simulink model "SWC_HALOUT_type"  (R2021b)
settings: Solver=FixedStepDiscrete  StartTime=0.0  StopTime=10.0  FixedStep=0.005  RelTol=1e-3
values from neighbouring files (symbols this model uses):
  DTC_10020B = Simulink.Parameter    [DTC_Constant_Definition.m]
  DTC_10020C = Simulink.Parameter    [DTC_Constant_Definition.m]
  DTC_10020D = Simulink.Parameter    [DTC_Constant_Definition.m]
  DTC_10020E = Simulink.Parameter    [DTC_Constant_Definition.m]
  DTC_100210 = Simulink.Parameter    [DTC_Constant_Definition.m]
  DTC_100211 = Simulink.Parameter    [DTC_Constant_Definition.m]
  DTC_100212 = Simulink.Parameter    [DTC_Constant_Definition.m]
  DTC_100213 = Simulink.Parameter    [DTC_Constant_Definition.m]
  DTC_100214 = Simulink.Parameter    [DTC_Constant_Definition.m]
  DTC_100215 = Simulink.Parameter    [DTC_Constant_Definition.m]
  DTC_100216 = Simulink.Parameter    [DTC_Constant_Definition.m]
  DTC_100217 = Simulink.Parameter    [DTC_Constant_Definition.m]
  DTC_100218 = Simulink.Parameter    [DTC_Constant_Definition.m]
  DTC_100219 = Simulink.Parameter    [DTC_Constant_Definition.m]
  DTC_10021A = Simulink.Parameter    [DTC_Constant_Definition.m]
  DTC_10021B = Simulink.Parameter    [DTC_Constant_Definition.m]
  DTC_10021C = Simulink.Parameter    [DTC_Constant_Definition.m]
  DTC_10021D = Simulink.Parameter    [DTC_Constant_Definition.m]
  DTC_10021E = Simulink.Parameter    [DTC_Constant_Definition.m]
  DTC_100220 = Simulink.Parameter    [DTC_Constant_Definition.m]
  DTC_100221 = Simulink.Parameter    [DTC_Constant_Definition.m]
  DTC_100223 = Simulink.Parameter    [DTC_Constant_Definition.m]
  DTC_100224 = Simulink.Parameter    [DTC_Constant_Definition.m]
  DTC_100225 = Simulink.Parameter    [DTC_Constant_Definition.m]
  DTC_100226 = Simulink.Parameter    [DTC_Constant_Definition.m]
  DTC_100227 = Simulink.Parameter    [DTC_Constant_Definition.m]
  DTC_100242 = Simulink.Parameter    [DTC_Constant_Definition.m]
  DTC_100243 = Simulink.Parameter    [DTC_Constant_Definition.m]
  DTC_100244 = Simulink.Parameter    [DTC_Constant_Definition.m]
  DTC_100247 = Simulink.Parameter    [DTC_Constant_Definition.m]
  DTC_100248 = Simulink.Parameter    [DTC_Constant_Definition.m]
  DTC_100249 = Simulink.Parameter    [DTC_Constant_Definition.m]
  DTC_100250 = Simulink.Parameter    [DTC_Constant_Definition.m]
  DTC_100251 = Simulink.Parameter    [DTC_Constant_Definition.m]
  DTC_100252 = Simulink.Parameter    [DTC_Constant_Definition.m]
  DTC_100A10 = Simulink.Parameter    [DTC_Constant_Definition.m]
  DTC_100A12 = Simulink.Parameter    [DTC_Constant_Definition.m]
  DTC_100A16 = Simulink.Parameter    [DTC_Constant_Definition.m]
  DTC_100A17 = Simulink.Parameter    [DTC_Constant_Definition.m]
  DTC_100A18 = Simulink.Parameter    [DTC_Constant_Definition.m]
  DTC_100A19 = Simulink.Parameter    [DTC_Constant_Definition.m]
  DTC_500B01 = Simulink.Parameter    [DTC_Constant_Definition.m]
  DTC_500B02 = Simulink.Parameter    [DTC_Constant_Definition.m]
  DTC_500B03 = Simulink.Parameter    [DTC_Constant_Definition.m]
  DTC_500B04 = Simulink.Parameter    [DTC_Constant_Definition.m]
  DTC_500B05 = Simulink.Parameter    [DTC_Constant_Definition.m]
  DTC_500B06 = Simulink.Parameter    [DTC_Constant_Definition.m]
  DTC_500B07 = Simulink.Parameter    [DTC_Constant_Definition.m]
  DTC_500B08 = Simulink.Parameter    [DTC_Constant_Definition.m]
  DTC_500B09 = Simulink.Parameter    [DTC_Constant_Definition.m]
  DTC_500B0A = Simulink.Parameter    [DTC_Constant_Definition.m]
  DTC_500B0B = Simulink.Parameter    [DTC_Constant_Definition.m]
  DTC_500B0C = Simulink.Parameter    [DTC_Constant_Definition.m]
  DTC_500B0D = Simulink.Parameter    [DTC_Constant_Definition.m]
  DTC_500B0E = Simulink.Parameter    [DTC_Constant_Definition.m]
  DTC_500B0F = Simulink.Parameter    [DTC_Constant_Definition.m]
  DTC_500B10 = Simulink.Parameter    [DTC_Constant_Definition.m]
  DTC_90021F = Simulink.Parameter    [DTC_Constant_Definition.m]
  DTC_90022F = Simulink.Parameter    [DTC_Constant_Definition.m]
  DTC_900253 = Simulink.Parameter    [DTC_Constant_Definition.m]
  DTC_900254 = Simulink.Parameter    [DTC_Constant_Definition.m]
  DTC_900301 = Simulink.Parameter    [DTC_Constant_Definition.m]
  DTC_900302 = Simulink.Parameter    [DTC_Constant_Definition.m]
  DTC_900303 = Simulink.Parameter    [DTC_Constant_Definition.m]
  DTC_900304 = Simulink.Parameter    [DTC_Constant_Definition.m]
  DTC_900305 = Simulink.Parameter    [DTC_Constant_Definition.m]
  DTC_900909 = Simulink.Parameter    [DTC_Constant_Definition.m]
  DTC_90090A = Simulink.Parameter    [DTC_Constant_Definition.m]
  DTC_90090B = Simulink.Parameter    [DTC_Constant_Definition.m]
  DTC_90090C = Simulink.Parameter    [DTC_Constant_Definition.m]
  DTC_90090D = Simulink.Parameter    [DTC_Constant_Definition.m]
  DTC_90090E = Simulink.Parameter    [DTC_Constant_Definition.m]
  DTC_90090F = Simulink.Parameter    [DTC_Constant_Definition.m]
  DTC_900910 = Simulink.Parameter    [DTC_Constant_Definition.m]
  DTC_900911 = Simulink.Parameter    [DTC_Constant_Definition.m]
  DTC_900912 = Simulink.Parameter    [DTC_Constant_Definition.m]
  DTC_900913 = Simulink.Parameter    [DTC_Constant_Definition.m]
  DTC_900914 = Simulink.Parameter    [DTC_Constant_Definition.m]
  DTC_C0288F = Simulink.Parameter    [DTC_Constant_Definition.m]
  DTC_C0378F = Simulink.Parameter    [DTC_Constant_Definition.m]
  DTC_C0468F = Simulink.Parameter    [DTC_Constant_Definition.m]
  DTC_C0558F = Simulink.Parameter    [DTC_Constant_Definition.m]
  DTC_C0648F = Simulink.Parameter    [DTC_Constant_Definition.m]
  DTC_C0808F = Simulink.Parameter    [DTC_Constant_Definition.m]
  DTC_D00201 = Simulink.Parameter    [DTC_Constant_Definition.m]
  DTC_D00202 = Simulink.Parameter    [DTC_Constant_Definition.m]
  DTC_D00203 = Simulink.Parameter    [DTC_Constant_Definition.m]
  DTC_D00204 = Simulink.Parameter    [DTC_Constant_Definition.m]
  DTC_D00205 = Simulink.Parameter    [DTC_Constant_Definition.m]
  DTC_D00206 = Simulink.Parameter    [DTC_Constant_Definition.m]
  DTC_D00207 = Simulink.Parameter    [DTC_Constant_Definition.m]
  DTC_D00208 = Simulink.Parameter    [DTC_Constant_Definition.m]
  DTC_D00209 = Simulink.Parameter    [DTC_Constant_Definition.m]
  DTC_D0020A = Simulink.Parameter    [DTC_Constant_Definition.m]
  DTC_D00228 = Simulink.Parameter    [DTC_Constant_Definition.m]
  DTC_D00229 = Simulink.Parameter    [DTC_Constant_Definition.m]
  DTC_D0022A = Simulink.Parameter    [DTC_Constant_Definition.m]
  DTC_D0022B = Simulink.Parameter    [DTC_Constant_Definition.m]
  DTC_D0022C = Simulink.Parameter    [DTC_Constant_Definition.m]
  DTC_D0022D = Simulink.Parameter    [DTC_Constant_Definition.m]
  DTC_D00230 = Simulink.Parameter    [DTC_Constant_Definition.m]
  DTC_D00231 = Simulink.Parameter    [DTC_Constant_Definition.m]
  DTC_D00232 = Simulink.Parameter    [DTC_Constant_Definition.m]
  DTC_D00234 = Simulink.Parameter    [DTC_Constant_Definition.m]
  DTC_D00235 = Simulink.Parameter    [DTC_Constant_Definition.m]
  DTC_D00236 = Simulink.Parameter    [DTC_Constant_Definition.m]
  DTC_D00237 = Simulink.Parameter    [DTC_Constant_Definition.m]
  DTC_D00238 = Simulink.Parameter    [DTC_Constant_Definition.m]
  DTC_D0023A = Simulink.Parameter    [DTC_Constant_Definition.m]
  DTC_D0023B = Simulink.Parameter    [DTC_Constant_Definition.m]
  DTC_D0023C = Simulink.Parameter    [DTC_Constant_Definition.m]
  DTC_D0023D = Simulink.Parameter    [DTC_Constant_Definition.m]
  DTC_D0023E = Simulink.Parameter    [DTC_Constant_Definition.m]
  DTC_D00240 = Simulink.Parameter    [DTC_Constant_Definition.m]
  DTC_D00241 = Simulink.Parameter    [DTC_Constant_Definition.m]
undefined symbols (not defined in the file or in its folder): DIDLen_APPD, DIDLen_APPE, DIDLen_APPPedalZP, DIDLen_APSFunConfig, DIDLen_AutoLock, DIDLen_AutoWipHSpdEN, DIDLen_CALID, DIDLen_CDEODT, DIDLen_CLRDIST, DIDLen_DKCBLESta, DIDLen_DKCKey, DIDLen_DKCSta, DIDLen_DoorNFCAnchorSta, DIDLen_DRLDis, DIDLen_DynoMode, DIDLen_ECUNAME, DIDLen_FDDKCCoordXY, DIDLen_FMHTimer, DIDLen_LFLowPresThre, DIDLen_LFSensorID, DIDLen_LIDAAnchorSta, DIDLen_LRLowPresThre, DIDLen_LRSensorID, DIDLen_MILDIST, DIDLen_NUMPSATRIPSFLTMEMCLR, DIDLen_NVMPedalZP, DIDLen_OBDReq, DIDLen_ODOMETER, DIDLen_PKE, DIDLen_ProtocolId, DIDLen_PSA, DIDLen_QTYPSATRIPS, DIDLen_RFLowPresThre, DIDLen_RFSensorID, DIDLen_RRLowPresThre, DIDLen_RRSensorID, DIDLen_RUNTM, DIDLen_SensorMode, DIDLen_TestGroup, DIDLen_TireSize, DIDLen_TPMSLearnSta, DIDLen_UIDSta, DIDLen_USSConfig, DIDLen_UWBAnchorSta, DIDLen_VIN, DIDLen_VSS, DIDLen_WhlPres, DIDLen_WhlSensorBattSta, DIDLen_WhlTmp, DIDLen_WipRLSCmdCutFilter, DIDLen_WipRLSCmdHoldFilter, DIDLen_XWDMode, DIDNum_APPD, DIDNum_APPE, DIDNum_APPPedalZP, DIDNum_APSFunConfig, DIDNum_AutoLock, DIDNum_AutoWipHSpdEN, DIDNum_CALID, DIDNum_CDEODT ... (+281)
libraries: simulink x213, FVT_lib x160, hdlsllib x6, hcu_lib x5, halout x1
(part 9 of 9)

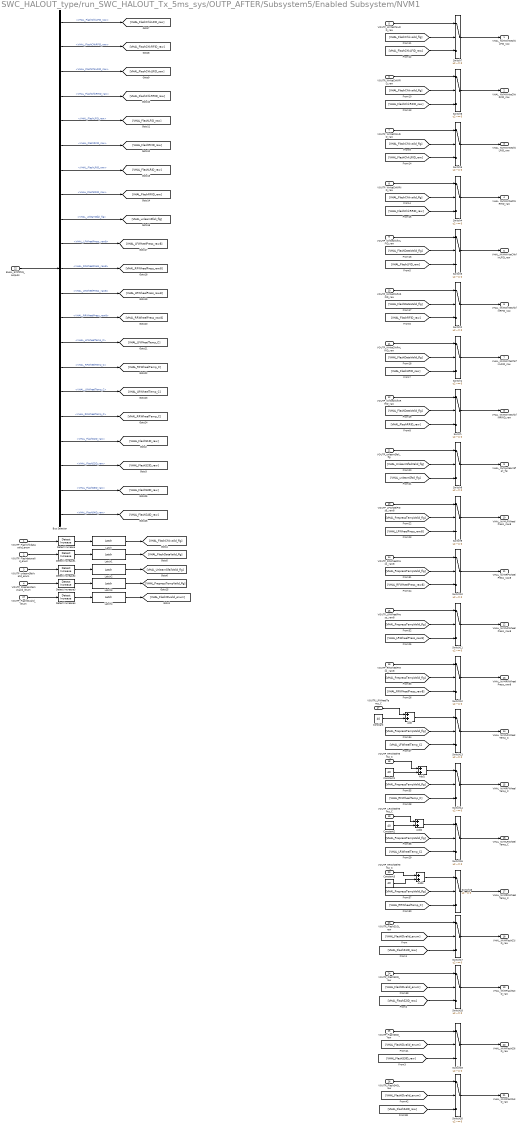
== system SWC_HALOUT_type/run_SWC_HALOUT_Tx_5ms_sys/OUTP_AFTER/Subsystem5/Enabled Subsystem/NVM1 ==
  VOUTP_Flashchkdatavalid_enum : Inport
  VOUTP_Flashdatavalid_enum : Inport  Port=2
  VOUTP_unlearnSfailvalid_enum : Inport  Port=3
  VOUTP_Prepresstempvalid_enum : Inport  Port=4
  VOUTP_WriteChkLFID_raw : Inport  Port=5
  VOUTP_WriteChkRFID_raw : Inport  Port=6
  VOUTP_WriteChkLRID_raw : Inport  Port=7
  VOUTP_WriteChkRRID_raw : Inport  Port=8
  VOUTP_WriteChkfinLFID_raw : Inport  Port=9
  VOUTP_WriteChkfinRFID_raw : Inport  Port=10
  VOUTP_WriteChkfinLRID_raw : Inport  Port=11
  VOUTP_WriteChkfinRRID_raw : Inport  Port=12
  VOUTP_LFWheelPress_raw8 : Inport  Port=13
  VOUTP_RFWheelPress_raw8 : Inport  Port=14
  VOUTP_LRWheelPress_raw8 : Inport  Port=15
  VOUTP_RRWheelPress_raw8 : Inport  Port=16
  VOUTP_LFWheelTemp_C : Inport  Port=17
  VOUTP_RFWheelTemp_C : Inport  Port=18
  VOUTP_LRWheelTemp_C : Inport  Port=19
  VOUTP_RRWheelTemp_C : Inport  Port=20
  VOUTP_unlearnSfali_flg : Inport  Port=21
  BHAL_SYSTPMS_outputs : Inport  Port=22
  VOUTP_FlashS1ID_raw : Inport  Port=23
  VOUTP_FlashS2ID_raw : Inport  Port=24
  VOUTP_FlashS3ID_raw : Inport  Port=25
  VOUTP_FlashS4ID_raw : Inport  Port=26
  VOUTP_FlashIDvalid_enum : Inport  Port=27
  Add{,1..3} (4 alike) : Sum
  Bus Selector : BusSelector  OutputSignals=VHAL_FlashChkLFID_raw,VHAL_FlashChkRFID_raw,VHAL_FlashChkLRID_raw,VHAL_FlashChkRRID_raw,VHAL_FlashLFID_raw,VHAL_FlashRFID_raw,VHAL_FlashLRID_raw,VHAL_FlashRRID_raw,VHAL_unlearnSfali_flg,VHAL_LFWheelPress_raw8,VHAL_RFWheelPress_raw8,VHAL_LRWheelPress_raw8,VHAL_RRWheelPress_raw8,VHAL_LFWheelTemp_C,VHAL_RFWheelTemp_C,VHAL_LRWheelTemp_C,VHAL_RRWheelTemp_C,VHAL_FlashS1ID_raw,VHAL_FlashS2ID_raw,VHAL_FlashS3ID_raw,VHAL_FlashS4ID_raw
  Constant{,1..3} (4 alike) : Constant  Value=40
  Detect Increase{,1..4} (5 alike) : simulink/Logic and Bit Operations/Detect Increase  vinit=0.0  OutDataTypeStr=boolean
  Latch{,1..4} (5 alike) : hcu_lib/Basic_Blocks/Latch
  Switch{,1..20} (21 alike) : Switch  Criteria=u2 ~= 0
  VHAL_NVMWriteChkLFID_raw : Outport
  VHAL_NVMWriteChkRFID_raw : Outport  Port=2
  VHAL_NVMWriteChkLRID_raw : Outport  Port=3
  VHAL_NVMWriteChkRRID_raw : Outport  Port=4
  VHAL_NVMWriteChkfinLFID_raw : Outport  Port=5
  VHAL_NVMWriteChkfinRFID_raw : Outport  Port=6
  VHAL_NVMWriteChkfinLRID_raw : Outport  Port=7
  VHAL_NVMWriteChkfinRRID_raw : Outport  Port=8
  VHAL_NVMunlearnSfali_flg : Outport  Port=9
  VHAL_NVMLFWheelPress_raw8 : Outport  Port=10
  VHAL_NVMRFWheelPress_raw8 : Outport  Port=11
  VHAL_NVMLRWheelPress_raw8 : Outport  Port=12
  VHAL_NVMRRWheelPress_raw8 : Outport  Port=13
  VHAL_NVMLFWheelTemp_C : Outport  Port=14
  VHAL_NVMRFWheelTemp_C : Outport  Port=15
  VHAL_NVMLRWheelTemp_C : Outport  Port=16
  VHAL_NVMRRWheelTemp_C : Outport  Port=17
  VHAL_NVMFlashS1ID_raw : Outport  Port=18
  VHAL_NVMFlashS2ID_raw : Outport  Port=19
  VHAL_NVMFlashS3ID_raw : Outport  Port=20
  VHAL_NVMFlashS4ID_raw : Outport  Port=21
  wires:
  Bus Selector/2 -> [VHAL_FlashChkRFID_raw]  "<VHAL_FlashChkRFID_raw>"
  Bus Selector/1 -> [VHAL_FlashChkLFID_raw]  "<VHAL_FlashChkLFID_raw>"
  Bus Selector/11 -> [VHAL_RFWheelPress_raw8]  "<VHAL_RFWheelPress_raw8>"
  Bus Selector/3 -> [VHAL_FlashChkLRID_raw]  "<VHAL_FlashChkLRID_raw>"
  Bus Selector/7 -> [VHAL_FlashLRID_raw]  "<VHAL_FlashLRID_raw>"
  Bus Selector/5 -> [VHAL_FlashLFID_raw]  "<VHAL_FlashLFID_raw>"
  Bus Selector/6 -> [VHAL_FlashRFID_raw]  "<VHAL_FlashRFID_raw>"
  Bus Selector/8 -> [VHAL_FlashRRID_raw]  "<VHAL_FlashRRID_raw>"
  Bus Selector/14 -> [VHAL_LFWheelTemp_C]  "<VHAL_LFWheelTemp_C>"
  Bus Selector/9 -> [VHAL_unlearnSfali_flg]  "<VHAL_unlearnSfali_flg>"
  Bus Selector/13 -> [VHAL_RRWheelPress_raw8]  "<VHAL_RRWheelPress_raw8>"
  Bus Selector/4 -> [VHAL_FlashChkRRID_raw]  "<VHAL_FlashChkRRID_raw>"
  Bus Selector/12 -> [VHAL_LRWheelPress_raw8]  "<VHAL_LRWheelPress_raw8>"
  BHAL_SYSTPMS_outputs/1 -> Bus Selector/1
  Bus Selector/15 -> [VHAL_RFWheelTemp_C]  "<VHAL_RFWheelTemp_C>"
  Bus Selector/10 -> [VHAL_LFWheelPress_raw8]  "<VHAL_LFWheelPress_raw8>"
  Bus Selector/17 -> [VHAL_RRWheelTemp_C]  "<VHAL_RRWheelTemp_C>"
  Bus Selector/16 -> [VHAL_LRWheelTemp_C]  "<VHAL_LRWheelTemp_C>"
  Switch/1 -> VHAL_NVMWriteChkfinRRID_raw/1
  Switch1/1 -> VHAL_NVMWriteChkfinLRID_raw/1
  Switch2/1 -> VHAL_NVMWriteChkfinRFID_raw/1
  Switch3/1 -> VHAL_NVMWriteChkfinLFID_raw/1
  Switch4/1 -> VHAL_NVMWriteChkRRID_raw/1
  Switch5/1 -> VHAL_NVMWriteChkLRID_raw/1
  Switch6/1 -> VHAL_NVMWriteChkRFID_raw/1
  Switch7/1 -> VHAL_NVMWriteChkLFID_raw/1
  Switch8/1 -> VHAL_NVMunlearnSfali_flg/1
  VOUTP_WriteChkRFID_raw/1 -> Switch6/1
  VOUTP_WriteChkLFID_raw/1 -> Switch7/1
  VOUTP_WriteChkfinLFID_raw/1 -> Switch3/1
  VOUTP_WriteChkRRID_raw/1 -> Switch4/1
  VOUTP_WriteChkLRID_raw/1 -> Switch5/1
  VOUTP_WriteChkfinRRID_raw/1 -> Switch/1
  VOUTP_WriteChkfinLRID_raw/1 -> Switch1/1
  [VHAL_FlashRRID_raw] -> Switch/3
  VOUTP_WriteChkfinRFID_raw/1 -> Switch2/1
  [VHAL_FlashChkvalid_flg] -> Switch7/2
  [VHAL_FlashChkvalid_flg] -> Switch4/2
  [VHAL_FlashRFID_raw] -> Switch2/3
  [VHAL_FlashLFID_raw] -> Switch3/3
  [VHAL_FlashChkLFID_raw] -> Switch7/3
  [VHAL_FlashChkLRID_raw] -> Switch5/3
  [VHAL_FlashDataValid_flg] -> Switch1/2
  [VHAL_FlashChkRRID_raw] -> Switch4/3
  [VHAL_FlashDataValid_flg] -> Switch/2
  [VHAL_FlashDataValid_flg] -> Switch3/2
  [VHAL_FlashChkvalid_flg] -> Switch5/2
  [VHAL_FlashDataValid_flg] -> Switch2/2
  [VHAL_FlashChkRFID_raw] -> Switch6/3
  [VHAL_FlashLRID_raw] -> Switch1/3
  [VHAL_FlashChkvalid_flg] -> Switch6/2
  VOUTP_Prepresstempvalid_enum/1 -> Detect Increase3/1
  VOUTP_unlearnSfailvalid_enum/1 -> Detect Increase2/1
  VOUTP_Flashdatavalid_enum/1 -> Detect Increase1/1
  VOUTP_Flashchkdatavalid_enum/1 -> Detect Increase/1
  Latch3/1 -> [VHAL_PrepressTempValid_flg]
  Detect Increase/1 -> Latch/1
  Detect Increase2/1 -> Latch2/1
  Latch1/1 -> [VHAL_FlashDataValid_flg]
  Latch2/1 -> [VHAL_UnlearnSfailValid_flg]
  Latch/1 -> [VHAL_FlashChkvalid_flg]
  Detect Increase3/1 -> Latch3/1
  Detect Increase1/1 -> Latch1/1
  [VHAL_unlearnSfali_flg] -> Switch8/3
  VOUTP_unlearnSfali_flg/1 -> Switch8/1
  [VHAL_UnlearnSfailValid_flg] -> Switch8/2
  VOUTP_RRWheelTemp_C/1 -> Add3/1
  VOUTP_LFWheelTemp_C/1 -> Add/1
  VOUTP_RFWheelTemp_C/1 -> Add1/1
  VOUTP_LRWheelTemp_C/1 -> Add2/1
  VOUTP_LFWheelPress_raw8/1 -> Switch9/1
  Switch16/1 -> VHAL_NVMRRWheelTemp_C/1
  Switch13/1 -> VHAL_NVMLFWheelTemp_C/1
  [VHAL_LRWheelTemp_C] -> Switch15/3
  Switch15/1 -> VHAL_NVMLRWheelTemp_C/1
  Switch14/1 -> VHAL_NVMRFWheelTemp_C/1
  [VHAL_PrepressTempValid_flg] -> Switch16/2
  VOUTP_RFWheelPress_raw8/1 -> Switch10/1
  Switch9/1 -> VHAL_NVMLFWheelPress_raw8/1
  Switch10/1 -> VHAL_NVMRFWheelPress_raw8/1
  [VHAL_LFWheelTemp_C] -> Switch13/3
  Switch11/1 -> VHAL_NVMLRWheelPress_raw8/1
  [VHAL_PrepressTempValid_flg] -> Switch9/2
  [VHAL_RFWheelTemp_C] -> Switch14/3
  [VHAL_RRWheelPress_raw8] -> Switch12/3
  Switch12/1 -> VHAL_NVMRRWheelPress_raw8/1
  [VHAL_PrepressTempValid_flg] -> Switch12/2
  [VHAL_PrepressTempValid_flg] -> Switch14/2
  [VHAL_LFWheelPress_raw8] -> Switch9/3
  [VHAL_LRWheelPress_raw8] -> Switch11/3
  [VHAL_RFWheelPress_raw8] -> Switch10/3
  [VHAL_PrepressTempValid_flg] -> Switch15/2
  VOUTP_LRWheelPress_raw8/1 -> Switch11/1
  [VHAL_PrepressTempValid_flg] -> Switch10/2
  [VHAL_RRWheelTemp_C] -> Switch16/3
  [VHAL_PrepressTempValid_flg] -> Switch13/2
  [VHAL_PrepressTempValid_flg] -> Switch11/2
  VOUTP_RRWheelPress_raw8/1 -> Switch12/1
  Detect Increase4/1 -> Latch4/1
  Latch4/1 -> [VHAL_FlashIDvalid_enum]
  VOUTP_FlashIDvalid_enum/1 -> Detect Increase4/1
  [VHAL_FlashS1ID_raw] -> Switch17/3
  [VHAL_FlashIDvalid_enum] -> Switch17/2
  Switch17/1 -> VHAL_NVMFlashS1ID_raw/1
  VOUTP_FlashS1ID_raw/1 -> Switch17/1
  Bus Selector/18 -> [VHAL_FlashS1ID_raw]  "<VHAL_FlashS1ID_raw>"
  Bus Selector/19 -> [VHAL_FlashS2ID_raw]  "<VHAL_FlashS2ID_raw>"
  Bus Selector/20 -> [VHAL_FlashS3ID_raw]  "<VHAL_FlashS3ID_raw>"
  Bus Selector/21 -> [VHAL_FlashS4ID_raw]  "<VHAL_FlashS4ID_raw>"
  [VHAL_FlashS2ID_raw] -> Switch18/3
  Switch18/1 -> VHAL_NVMFlashS2ID_raw/1
  VOUTP_FlashS2ID_raw/1 -> Switch18/1
  [VHAL_FlashIDvalid_enum] -> Switch18/2
  Switch19/1 -> VHAL_NVMFlashS3ID_raw/1
  [VHAL_FlashS3ID_raw] -> Switch19/3
  [VHAL_FlashIDvalid_enum] -> Switch19/2
  VOUTP_FlashS3ID_raw/1 -> Switch19/1
  Switch20/1 -> VHAL_NVMFlashS4ID_raw/1
  [VHAL_FlashS4ID_raw] -> Switch20/3
  [VHAL_FlashIDvalid_enum] -> Switch20/2
  VOUTP_FlashS4ID_raw/1 -> Switch20/1
  Constant/1 -> Add/2
  Add/1 -> Switch13/1
  Add1/1 -> Switch14/1
  Constant1/1 -> Add1/2
  Add2/1 -> Switch15/1
  Constant2/1 -> Add2/2
  Add3/1 -> Switch16/1
  Constant3/1 -> Add3/2

== system SWC_HALOUT_type/run_SWC_HALOUT_Tx_5ms_sys/OUTP_AFTER/Subsystem5/Enabled Subsystem/Subsystem ==
  VOUTP_DiagFMHT_s : Inport
  Add1 : Sum  Inputs=+-
  Constant45 : Constant  Value=10
  Gain4 : Gain  Gain=1/5
  Saturation : Saturate  UpperLimit=150  LowerLimit=5
  Out1 : Outport
  wires:
  VOUTP_DiagFMHT_s/1 -> Add1/1
  Constant45/1 -> Add1/2
  Gain4/1 -> Out1/1
  Saturation/1 -> Gain4/1
  Add1/1 -> Saturation/1

== stateflow chart SWC_HALOUT_type/run_SWC_HALOUT_Tx_5ms_sys/hcu_main_sched ==
  state Main_Scheduler
    (default) -> (junction 31) : {
        |   Sys_Init_done = FALSE;
        |   trig_Read_NVM_00;
        |   trig_ReadIMUOffset_00;
        | }
    Main_Scheduler -> (junction 31) : {Sys_Init_done = TRUE;}
    (junction 31) -> (junction 34) [order 1] : [
        |    Sys_Init_done &&...
        |    !VHAL_FusionSchedReq_flg
        | ]
    (junction 31) -> (junction 38) [order 2]
    (junction 34) -> (junction 36) : {
        |     trig_WDG;
        |     trig_GetNMID;
        |     trig_GetDID;
        |     trig_HAL_IN_10;
        |     trig_HAL_CDD_10_1;
        |     trig_HAL_DKC_10_2;
        |     trig_HAL_DKC_10_3;
        |     trig_INP_20;
        |     trig_APP_30;
        |     trig_OUTP_40;
        |     trig_OUTP_AFTER_40_1;
        |     trig_SetDID;
        |     trig_HAL_OUT_50;
        |     trig_HAL_OUTAFTER_50_1;
        |    }
    (junction 36) -> (junction 38)
  (default) -> Main_Scheduler
  data: VHAL_FusionSchedReq_flg input; Sys_Init_done local double; FALSE parameter; TRUE parameter
  events: trig_Read_NVM_00 output FUNCTION_CALL_EVENT; trig_ReadIMUOffset_00 output FUNCTION_CALL_EVENT; trig_WDG output FUNCTION_CALL_EVENT; trig_GetNMID output FUNCTION_CALL_EVENT; trig_GetDID output FUNCTION_CALL_EVENT; trig_HAL_IN_10 output FUNCTION_CALL_EVENT; trig_HAL_CDD_10_1 output FUNCTION_CALL_EVENT; trig_HAL_DKC_10_2 output FUNCTION_CALL_EVENT; trig_HAL_DKC_10_3 output FUNCTION_CALL_EVENT; trig_INP_20 output FUNCTION_CALL_EVENT; trig_APP_30 output FUNCTION_CALL_EVENT; trig_OUTP_40 output FUNCTION_CALL_EVENT; trig_OUTP_AFTER_40_1 output FUNCTION_CALL_EVENT; trig_SetDID output FUNCTION_CALL_EVENT; trig_HAL_OUT_50 output FUNCTION_CALL_EVENT; trig_HAL_OUTAFTER_50_1 output FUNCTION_CALL_EVENT
